simulink model "DC_motor_PM_SE"  (R2023a)
settings: Solver=VariableStepAuto  StartTime=0.0  StopTime=10  RelTol=1e-3  EnableMultiTasking=on
libraries: spsGroundLib x4, spsDCVoltageSourceLib x3, spsDCMachineLib x2, sps_lib x2, spsCurrentMeasurementLib x2
settings Model: Creator=Douglas  LastModifiedBy=Admin
settings SolverCC: AlgebraicLoopSolver=TrustRegion
settings DataIOCC: ReturnWorkspaceOutputs=off
settings OptimizationCC: LifeSpan=inf
settings DebuggingCC: UnconnectedInputMsg=warning  UnconnectedOutputMsg=warning  UnconnectedLineMsg=warning  SFUnexpectedBacktrackingDiag=warning  SFNoUnconditionalDefaultTransitionDiag=warning  ArithmeticOperatorsInVariantConditions=warning
settings ModelReferenceCC: EnableRefExpFcnMdlSchedulingChecks=on
settings SFSimCC: SimUseLocalCustomCode=off  CustomCodeUndefinedFunction=UseInterfaceOnly
settings RTWCC: RTWUseLocalCustomCode=off
settings CodeAppCC: StateflowObjectComments=on
settings GRTTargetCC: TargetLangStandard=C89/C90 (ANSI)
settings ConfigComp: CovMetricSettings=dw  CovSaveCumulativeToWorkspaceVar=on  CovSaveSingleToWorkspaceVar=on  CovExternalEMLEnable=off
settings SimscapeCC: SimscapeNormalizeSystem=off

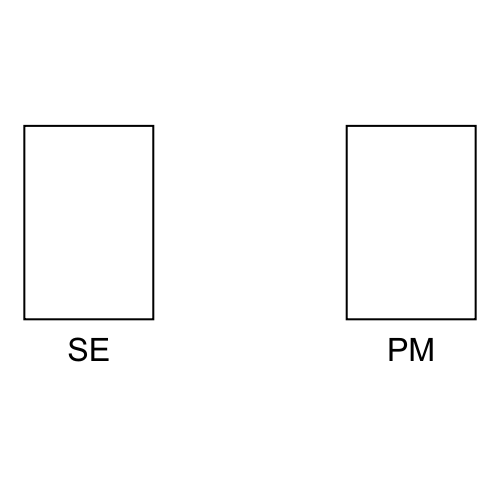
[thumbnail: Simulink's stored preview of the top-level diagram]
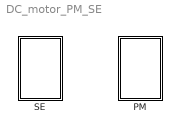
== system DC_motor_PM_SE ==
  PM : Subsystem
  SE : Subsystem

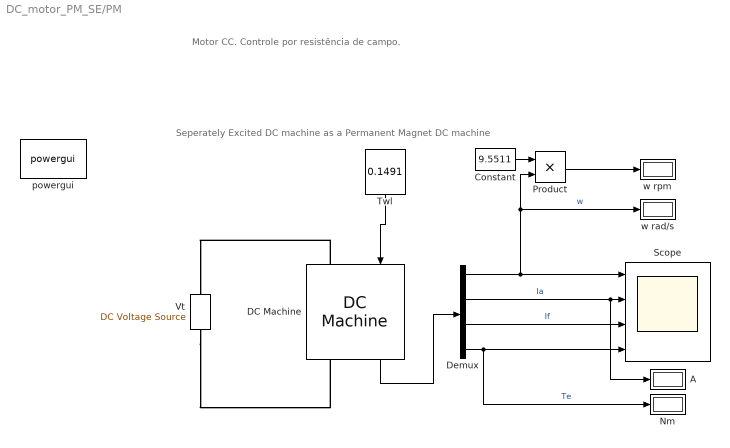
== system DC_motor_PM_SE/PM ==
  note: Seperately Excited DC machine as a Permanent Magnet DC machine
  note: Motor CC. Controle por resistência de campo.
  A : Display
  Constant : Constant  Value=9.5511
  DC Machine : spsDCMachineLib/DC Machine  PresetModel=No  MechanicalLoad=Torque TL  FieldType=Permanent magnet  ShowDetailedParameters=on  MeasurementBus=off  RLa=[ 3.09 0.055]  RLf="[ 2.02  0.27]"  Laf=0.12  MachineConstant=Back-emf constant (V/rpm)  Ke=0.029  Kt=0.2758  J=0.013  Bm=0.00063  Tf=0.0958  w0=0  Ifinit=2.47524752475248  TsPowergui=0  TsBlock=-1
  Demux : Demux
  Nm : Display
  Product : Product
  Scope : Scope  NumInputPorts=4
  Twl : Constant  Value=0.1491
  Vt : spsDCVoltageSourceLib/DC Voltage Source  Amplitude=80  Measurements=None
  powergui : sps_lib/powergui  Priority=1  SimulationMode=Continuous  SampleTime=50e-6  frequency=60  Iterations=50  frequencyindice=0  Pbase=100e6  ErrMax=1e-4  UnitsV=kV  UnitsW=MW  buscounter=0  FunctionMessages=off  echomessages=off  EnableUseOfTLC=off  CurrentSourceSwitches=off  DisableSnubberDevices=off  DisableRonSwitches=off  DisableVfSwitches=off  DisplayEquations=off  AutomaticDiscreteSolvers=off  SolverType=Tustin/Backward Euler (TBE)  Interpol=off  ExternalGateDelay=off  methode=off  Ts=10  x0status=blocks  SPID=off  SwTol=0  HookPort=off  NonlinearTolerance=1e-4  nMaxIteration=100  ContinueOnMaxIteration=off  RestoreLinks=warning  ResistiveCurrentMeasurement=off  Frange=[0:2:500]  Ylog=off  Xlog=on  ShowGrid=off  save=off  variable=ZData  structure=0  ZoomFFT=off  StartTime=0.0  cycles=1  DisplayStyle=1  fundamental=60  FreqAxis=off  MaxFrequency=1000  frequencyindicesteady=1  RmsSteady=1  display=off
  w rad/s : Display
  w rpm : Display
  wires:
  Twl/1 -> DC Machine/1
  Constant/1 -> Product/1
  Demux/1 -> Scope/1, w rad/s/1, Product/2  "w"
  Demux/4 -> Scope/4, Nm/1  "Te"
  Demux/3 -> Scope/3  "If"
  Demux/2 -> A/1, Scope/2  "Ia"
  DC Machine/1 -> Demux/1
  Product/1 -> w rpm/1
  connections:
  Vt/LConn1 -- DC Machine/RConn1
  DC Machine/LConn1 -- Vt/RConn1

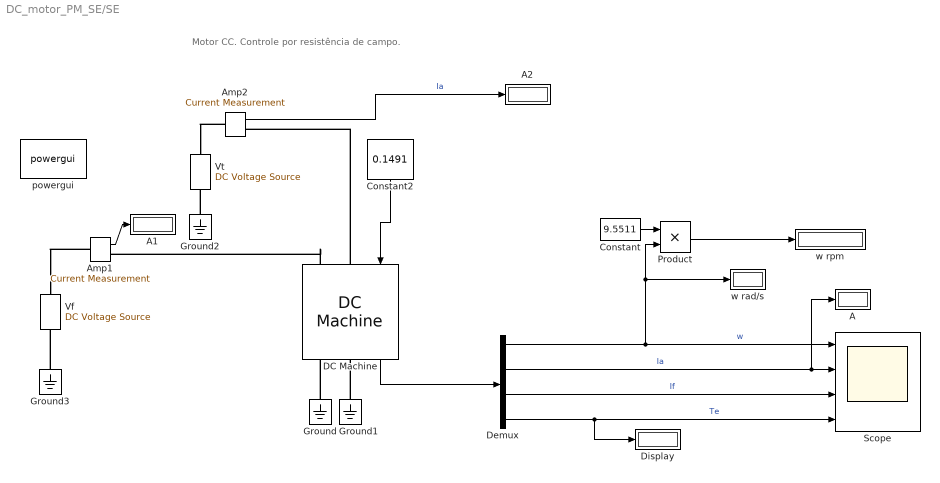
== system DC_motor_PM_SE/SE ==
  note: Motor CC. Controle por resistência de campo.
  A : Display
  A1 : Display
  A2 : Display
  Amp1 : spsCurrentMeasurementLib/Current Measurement  PhasorSimulation=off  OutputType=Complex  PSBequivalent=0
  Amp2 : spsCurrentMeasurementLib/Current Measurement  PhasorSimulation=off  OutputType=Complex  PSBequivalent=0
  Constant : Constant  Value=9.5511
  Constant2 : Constant  Value=0.1491
  DC Machine : spsDCMachineLib/DC Machine  PresetModel=No  MechanicalLoad=Torque TL  FieldType=Wound  ShowDetailedParameters=on  MeasurementBus=off  RLa="[ 3.09  0.055]"  RLf="[ 2.02  0.27]"  Laf=0.11  MachineConstant=Torque constant (N.m/A)  Ke=1.8  Kt=1.8  J=0.013  Bm=0.00063  Tf=0.0958  w0=0  Ifinit=2.50990099009901  TsPowergui=0  TsBlock=-1
  Demux : Demux
  Display : Display
  Ground{,1..3} (4 alike) : spsGroundLib/Ground  LConnTagsString=a
  Product : Product
  Scope : Scope  NumInputPorts=4
  Vf : spsDCVoltageSourceLib/DC Voltage Source  Amplitude=5.07  Measurements=None
  Vt : spsDCVoltageSourceLib/DC Voltage Source  Amplitude=80  Measurements=None
  powergui : sps_lib/powergui  Priority=1  SimulationMode=Continuous  SampleTime=50e-6  frequency=60  Iterations=50  frequencyindice=0  Pbase=100e6  ErrMax=1e-4  UnitsV=kV  UnitsW=MW  buscounter=0  FunctionMessages=off  echomessages=off  EnableUseOfTLC=off  CurrentSourceSwitches=off  DisableSnubberDevices=off  DisableRonSwitches=off  DisableVfSwitches=off  DisplayEquations=off  AutomaticDiscreteSolvers=off  SolverType=Tustin/Backward Euler (TBE)  Interpol=off  ExternalGateDelay=off  methode=off  Ts=10  x0status=blocks  SPID=off  SwTol=0  HookPort=off  NonlinearTolerance=1e-4  nMaxIteration=100  ContinueOnMaxIteration=off  RestoreLinks=warning  ResistiveCurrentMeasurement=off  Frange=[0:2:500]  Ylog=off  Xlog=on  ShowGrid=off  save=off  variable=ZData  structure=0  ZoomFFT=off  StartTime=0.0  cycles=1  DisplayStyle=1  fundamental=60  FreqAxis=off  MaxFrequency=1000  frequencyindicesteady=1  RmsSteady=1  display=off
  w rad/s : Display
  w rpm : Display
  wires:
  Amp1/1 -> A1/1
  Product/1 -> w rpm/1
  DC Machine/1 -> Demux/1
  Demux/2 -> A/1, Scope/2  "Ia"
  Demux/3 -> Scope/3  "If"
  Demux/4 -> Scope/4, Display/1  "Te"
  Demux/1 -> w rad/s/1, Product/2, Scope/1  "w"
  Constant/1 -> Product/1
  Amp2/1 -> A2/1  "Ia"
  Constant2/1 -> DC Machine/1
  connections:
  Ground/LConn1 -- DC Machine/RConn2
  Ground3/LConn1 -- Vf/LConn1
  Amp2/LConn1 -- Vt/RConn1
  Ground2/LConn1 -- Vt/LConn1
  Ground1/LConn1 -- DC Machine/RConn1
  Amp1/LConn1 -- Vf/RConn1
  DC Machine/LConn2 -- Amp1/RConn1
  DC Machine/LConn1 -- Amp2/RConn1
